simulink model "testehibrido"  (R2019a)
settings: Solver=FixedStepAuto  StartTime=0.0  StopTime=15.0  FixedStep=sampleTime  RelTol=1e-3
values from neighbouring files (symbols this model uses):
  FIR = FIR_Standard    [Lab_3.m]
settings Model: Creator=w  LastModifiedBy=w

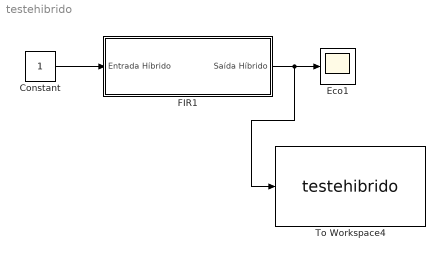
== system testehibrido ==
  Constant : Constant  SampleTime=1
  Eco1 : Scope
  FIR1 : Subsystem
  To Workspace4 : ToWorkspace  VariableName=testehibrido  SaveFormat=Structure With Time  SampleTime=-1
  wires:
  Constant/1 -> FIR1/1(Entrada Híbrido)
  FIR1/1(Saída Híbrido) -> To Workspace4/1, Eco1/1

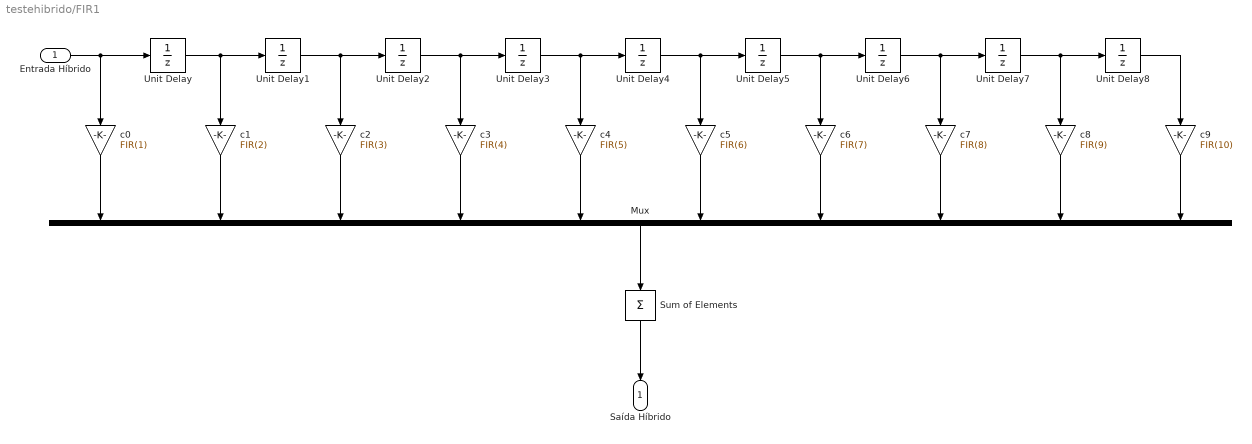
== system testehibrido/FIR1 ==
  Entrada Híbrido : Inport
  Mux : Mux  Inputs=10
  Sum of Elements : Sum  Inputs=+
  Unit Delay{,1..8} (9 alike) : UnitDelay  SampleTime=-1  HasFrameUpgradeWarning=on
  c0 : Gain  Gain=FIR(1)
  c1 : Gain  Gain=FIR(2)
  c2 : Gain  Gain=FIR(3)
  c3 : Gain  Gain=FIR(4)
  c4 : Gain  Gain=FIR(5)
  c5 : Gain  Gain=FIR(6)
  c6 : Gain  Gain=FIR(7)
  c7 : Gain  Gain=FIR(8)
  c8 : Gain  Gain=FIR(9)
  c9 : Gain  Gain=FIR(10)
  Saída Híbrido : Outport
  wires:
  Unit Delay1/1 -> c2/1, Unit Delay2/1
  Entrada Híbrido/1 -> Unit Delay/1, c0/1
  Unit Delay/1 -> Unit Delay1/1, c1/1
  Unit Delay2/1 -> c3/1, Unit Delay3/1
  Unit Delay7/1 -> c8/1, Unit Delay8/1
  Unit Delay8/1 -> c9/1
  Unit Delay5/1 -> Unit Delay6/1, c6/1
  Unit Delay6/1 -> c7/1, Unit Delay7/1
  Unit Delay4/1 -> Unit Delay5/1, c5/1
  Unit Delay3/1 -> Unit Delay4/1, c4/1
  Mux/1 -> Sum of Elements/1
  Sum of Elements/1 -> Saída Híbrido/1
  c0/1 -> Mux/1
  c1/1 -> Mux/2
  c9/1 -> Mux/10
  c8/1 -> Mux/9
  c7/1 -> Mux/8
  c6/1 -> Mux/7
  c5/1 -> Mux/6
  c4/1 -> Mux/5
  c3/1 -> Mux/4
  c2/1 -> Mux/3
